simulink model "motor_model_v1"  (R2016a)
settings: Solver=VariableStepAuto  StartTime=0.0  StopTime=1  RelTol=1e-3
values from neighbouring files (symbols this model uses):
  D = Dmotor + (Nm / No)^2 * (Dgearbox + Dexternal)    (= 0.005)    [load_motor_params.m]    (also in motor_params_latest.mat)
  J = Jmotor + (Nm / No)^2 * (Jgearbox + Jexternal)    (= 1.4200031758e-05)    [load_motor_params.m]    (also in motor_params_latest.mat)
  Kt = 30.2 * 1e-3    (= 0.0302)    [load_motor_params.m]    (also in motor_params_latest.mat)
  Kv = (1/317) * 60/(2*pi)    (= 0.0301239639922)    [load_motor_params.m]    (also in motor_params_latest.mat)
  La = 0.082 * 1e-3    (= 8.2e-05)    [load_motor_params.m]    (also in motor_params_latest.mat)
  Nm = 1    [load_motor_params.m]    (also in motor_params_latest.mat)
  No = 230    [load_motor_params.m]    (also in motor_params_latest.mat)
  Ra = 0.299    [load_motor_params.m]    (also in motor_params_latest.mat)
settings Model: Creator=user  LastModifiedBy=user

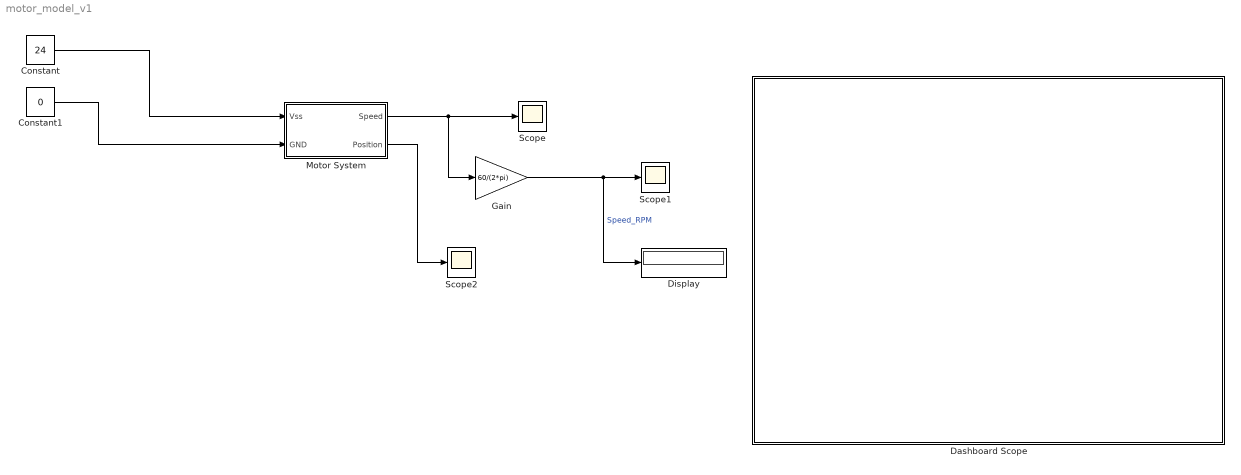
== system motor_model_v1 ==
  Constant : Constant  Value=24
  Constant1 : Constant  Value=0
  Dashboard Scope : Subsystem  DialogController=hmiCreateDDGDialog  IsWebBlock=on  mask(MWDashboardBlock){webBlockId=ecdd70a7-2b72-4acf-bca9-833aaf066668, webBlockType=sdiscope, ShowInitialText=on, HMISrcModelName=motor_model_v1}
      mask prompts: webBlockId "WebBlock Id"; webBlockType "WebBlock Type"; HMISrcModelName "Source Model"
      mask Help: helpview([docroot '/mapfiles/simulink.map'], 'hmi_scope')
      mask Display:
      | if strcmp(get_param(bdroot(gcb),'BlockDiagramType'), 'library')
      |     image([(matlabroot) '/toolbox/simulink/hmi/icons/DashboardScope.png']);
      | end
  Display : Display
      settings: Decimation=4
  Gain : Gain  Gain=60/(2*pi)
  Motor System : Subsystem
  Scope : Scope
  Scope1 : Scope
  Scope2 : Scope
  wires:
  Constant1/1 -> Motor System/2(GND)
  Motor System/1(Speed) -> Gain/1, Scope/1
  Gain/1 -> Display/1, Scope1/1  "Speed_RPM"
  Motor System/2(Position) -> Scope2/1
  Constant/1 -> Motor System/1(Vss)

== system motor_model_v1/Dashboard Scope ==

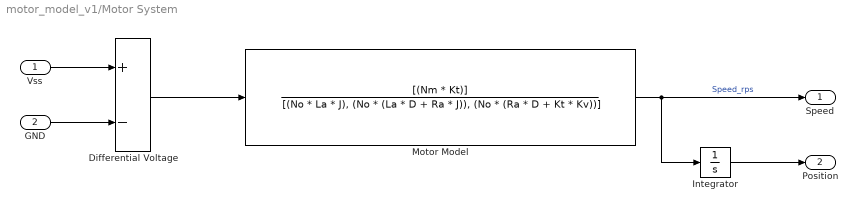
== system motor_model_v1/Motor System ==
  Vss : Inport
  GND : Inport  Port=2
  Differential Voltage : Sum  Inputs=+-
  Integrator : Integrator
  Motor Model : TransferFcn  Numerator=[(Nm * Kt)]  Denominator=[(No * La * J), (No * (La * D + Ra * J)), (No * (Ra * D + Kt * Kv))]
  Speed : Outport
  Position : Outport  Port=2
  wires:
  Differential Voltage/1 -> Motor Model/1
  Vss/1 -> Differential Voltage/1
  GND/1 -> Differential Voltage/2
  Motor Model/1 -> Integrator/1, Speed/1  "Speed_rps"
  Integrator/1 -> Position/1
